simulink model "ObservadorPlantaReal"  (R2016a)
settings: Solver=ode3  SolverMode=SingleTasking  StartTime=0.0  StopTime=10  RelTol=1e-3
values from neighbouring files (symbols this model uses):
  A = [0 1; -Mt/I -Kf/I]    [HinfPlantSeguroa.m]    (also in HinfPlanta.m)
  B = [0; L1/I]    [HinfPlantSeguroa.m]    (also in HinfPlanta.m)
  C = [1 0]    [HinfPlantSeguroa.m]    (also in HinfPlanta.m)
  L = G1*K1    [HinfPlantSeguroa.m]    (also in HinfPlanta.m)
libraries: arduino_io_lib x5
settings Model: FPTRunName=Active  ExtModeTrigDuration=2  Creator=The MathWorks, Inc.  LastModifiedBy=i95sa
settings DataIOCC: LimitDataPoints=on  SaveFormat=Array
settings OptimizationCC: DefaultParameterBehavior=Inlined  ExpressionDepthLimit=2147483647  OptimizeModelRefInitCode=on  LifeSpan=Inf  MaxStackSize=64
settings DebuggingCC: UnderspecifiedInitializationDetection=Classic  MergeDetectMultiDrivingBlocksExec=none  ParameterOverflowMsg=warning  FcnCallInpInsideContextMsg=EnableAllAsWarning  AllowSymbolicDim=off  StateNameClashWarn=warning
settings HardwareCC: UseEmbeddedCoderFeatures=off  UseSimulinkCoderFeatures=off
settings ModelReferenceCC: PropagateSignalLabelsOutOfModel=off
settings RTWCC: SystemTargetFile=ert.tlc  TemplateMakefile=ert_default_tmf  GenerateReport=on  RTWVerbose=off  Toolchain=Arduino AVR v1.6.1  BuildConfiguration=Faster Runs  LaunchReport=on
settings CodeAppCC: ForceParamTrailComments=on  IgnoreCustomStorageClasses=off  OperatorAnnotations=on  SimulinkDataObjDesc=on  SFDataObjDesc=on  MATLABFcnDesc=on  CustomSymbolStrType=$N$R$M  InsertBlockDesc=on  MATLABSourceComments=on  InternalIdentifier=Classic
settings ERTTargetCC: SupportNonInlinedSFcns=on  ERTCustomFileTemplate=example_file_process.tlc
settings ConfigComp: CovSFcnEnable=off

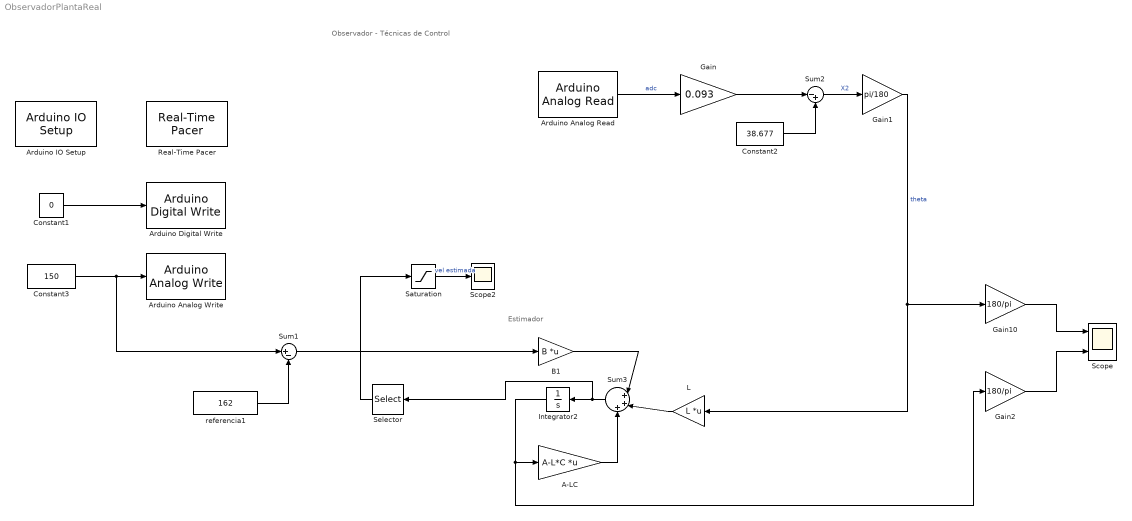
== system ObservadorPlantaReal ==
  note: Observador - Técnicas de Control
  note: Estimador
  A-LC : Gain  Gain=A-L*C  Multiplication=Matrix(K*u)
  Arduino Analog Read : arduino_io_lib/Arduino Analog Read  arduinoVar=Existing workspace arduino variable #1  arduinoPin=8  T=0.1
  Arduino Analog Write : arduino_io_lib/Arduino Analog Write  arduinoVar=Existing workspace arduino variable #1  arduinoPin=3  T=0.1
  Arduino Digital Write : arduino_io_lib/Arduino Digital Write  arduinoVar=Existing workspace arduino variable #1  arduinoPin=12  T=0.1
  Arduino IO Setup : arduino_io_lib/Arduino IO Setup  Priority=3  arduinoVar=Existing workspace arduino variable #1  workspaceVarName=ard  comPort=4
  B1 : Gain  Gain=B  Multiplication=Matrix(K*u)
  Constant1 : Constant  Value=0
  Constant2 : Constant  Value=38.677
  Constant3 : Constant  Value=150
  Gain : Gain  Gain=0.093
  Gain1 : Gain  Gain=pi/180
  Gain10 : Gain  Gain=180/pi
  Gain2 : Gain  Gain=180/pi
  Integrator2 : Integrator
  L : Gain  Gain=L  Multiplication=Matrix(K*u)
  Real-Time Pacer : arduino_io_lib/Real-Time Pacer  simTimePerRealTime=1
  Saturation : Saturate  UpperLimit=inf  LowerLimit=-1
  Scope : Scope  NumInputPorts=2
  Scope2 : Scope
  Selector : Selector  InputPortWidth=2  IndexOptions=Index vector (dialog)  Indices=[1]  OutputSizes=1
  Sum1 : Sum  Inputs=|+-
  Sum2 : Sum  Inputs=|-+
  Sum3 : Sum  Inputs=|+++
  referencia1 : Constant  Value=162
  wires:
  Arduino Analog Read/1 -> Gain/1  "adc"
  Constant1/1 -> Arduino Digital Write/1
  Gain/1 -> Sum2/1
  Constant2/1 -> Sum2/2
  Sum2/1 -> Gain1/1  "X2"
  Gain2/1 -> Scope/2
  Gain10/1 -> Scope/1
  Gain1/1 -> L/1, Gain10/1  "theta"
  Saturation/1 -> Scope2/1  "vel estimada"
  Constant3/1 -> Sum1/1, Arduino Analog Write/1
  B1/1 -> Sum3/1
  Integrator2/1 -> A-LC/1, Gain2/1
  A-LC/1 -> Sum3/3
  L/1 -> Sum3/2
  Sum3/1 -> Selector/1, Integrator2/1
  Selector/1 -> Saturation/1
  referencia1/1 -> Sum1/2
  Sum1/1 -> B1/1
